simulink model "Pendulo"  (R2020b)
settings: Solver=FixedStepAuto  StartTime=0.0  StopTime=180  FixedStep=0.05  RelTol=1e-3
values from neighbouring files (symbols this model uses):
  g = 9.81    [PIDMiplanta.m]    (also in PID_Pendulo.m)
  l = 1.5    [PIDMiplanta.m]    (also in PID_Pendulo.m = 6.096)
  M = 583.756    [PIDMiplanta.m]    (also in PID_Pendulo.m)
  m = 116.7512    [PIDMiplanta.m]    (also in PID_Pendulo.m)
libraries: pid_lib x2, dspsrcs4 x1, commchan3 x1
settings Model: Creator=Matias  LastModifiedBy=Matias

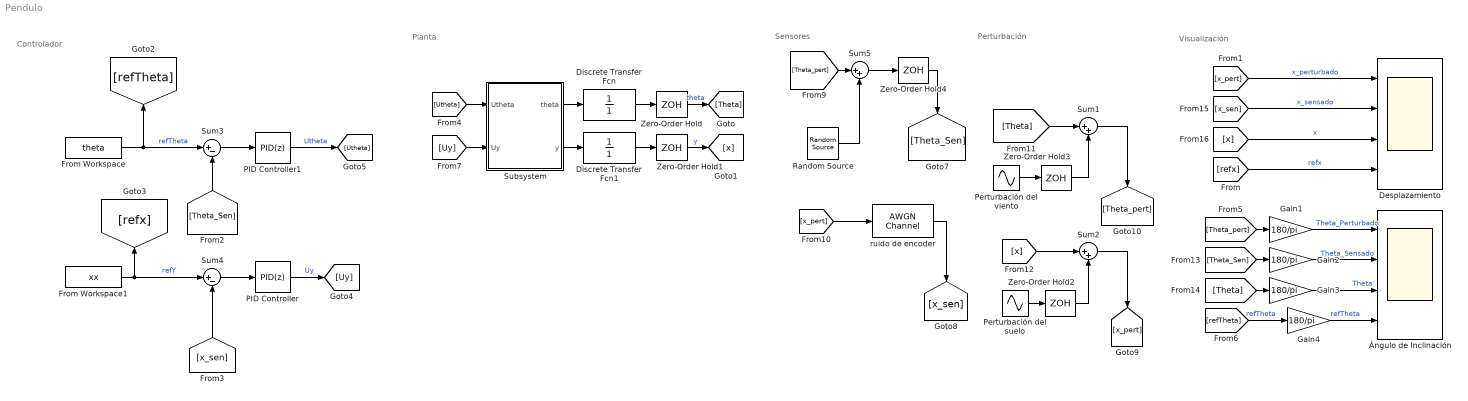
== system Pendulo ==
  note: Controlador
  note: Planta
  note: Perturbación
  note: Sensores
  note: Visualización
  Desplazamiento : Scope  NumInputPorts=4
  Discrete Transfer Fcn : DiscreteTransferFcn  Denominator=[1]
  Discrete Transfer Fcn1 : DiscreteTransferFcn  Denominator=[1]
  From Workspace : FromWorkspace  VariableName=theta
  From Workspace1 : FromWorkspace  VariableName=xx
  Gain{1..4} (4 alike) : Gain  Gain=180/pi
  PID Controller : pid_lib/PID Controller  Controller=PID  Form=Parallel  TimeDomain=Discrete-time  UseExternalTs=off  SampleTime=-1  IntegratorMethod=Forward Euler  FilterMethod=Forward Euler  ControllerParametersSource=internal  P=367.793686927  I=26.4785457931426  D=1277.18679492305  UseFilter=off  N=995.361556715437  TunerSelectOption=Transfer Function Based (PID Tuner App)  InitialConditionSource=internal  InitialConditionForIntegrator=0  InitialConditionForFilter=0  DifferentiatorICPrevScaledInput=0  ExternalReset=none  TrackingMode=off  Kt=1  LimitOutput=off  SatLimitsSource=internal  UpperSaturationLimit=inf  LowerSaturationLimit=-inf  LinearizeAsGain=on  AntiWindupMode=none  Kb=1  POutMin=[]  POutMax=[]  IOutMin=[]  IOutMax=[]  DOutMin=[]  DOutMax=[]  NOutMin=[]  NOutMax=[]  SumOutMin=[]  SumOutMax=[]  SaturationOutMin=[]  SaturationOutMax=[]  PParamMin=[]  PParamMax=[]  IParamMin=[]  IParamMax=[]  DParamMin=[]  DParamMax=[]  NParamMin=[]  NParamMax=[]  KbParamMin=[]  KbParamMax=[]  KtParamMin=[]  KtParamMax=[]  KbOutMin=[]  KbOutMax=[]  KtOutMin=[]  KtOutMax=[]  IntegratorOutMin=[]  IntegratorOutMax=[]  FilterOutMin=[]  FilterOutMax=[]  SumI1OutMin=[]  SumI1OutMax=[]  SumI2OutMin=[]  SumI2OutMax=[]  SumI3OutMin=[]  SumI3OutMax=[]  SumI4OutMin=[]  SumI4OutMax=[]  SumDOutMin=[]  SumDOutMax=[]  DifferentiatorOutMin=[]  DifferentiatorOutMax=[]  FilterDiffOutCoefMin=[]  FilterDiffOutCoefMax=[]  ReciprocalOutMin=[]  ReciprocalOutMax=[]  SumDenOutMin=[]  SumDenOutMax=[]  SumNumOutMin=[]  SumNumOutMax=[]  DivideOutMin=[]  DivideOutMax=[]  UdiffTsProdOutMin=[]  UdiffTsProdOutMax=[]  NTsProdOutMin=[]  NTsProdOutMax=[]  UintegralTsProdOutMin=[]  UintegralTsProdOutMax=[]  UngainTsProdOutMin=[]  UngainTsProdOutMax=[]  IntegratorContinuousStateAttributes=''  IntegratorStateMustResolveToSignalObject=off  IntegratorRTWStateStorageClass=Auto  FilterContinuousStateAttributes=''  FilterStateMustResolveToSignalObject=off  FilterRTWStateStorageClass=Auto  ParallelPVariant=InternalParameters  IdealPVariant=Disabled  IVariant=InternalParameters  DVariant=InternalParameters  IntegratorVariant=Discrete  SatVariant=Disabled  AWVariant=Passthrough  PCopyVariant=Disabled  TRVariant=Disabled  FdbkBlocksVariant=Forward  IdealPFdbkVariant=Disabled  SatFdbkVariant=Disabled  DerivativeFilterVariant=Differentiator  NVariant=Passthrough  NCopyVariant=Disabled_SignalSpec  FilterICVariant=InternalICsDifferentiator  IntegratorICVariant=InternalICs  ExternalResetVariant=Disabled  TRSumVariant=Passthrough  SumFdbkVariant=Disabled  SumVariant=Sum_PID  TsampFilterVariant=InternalTs  TsampNgainVariant=Passthrough  TsampIntegralVariant=Passthrough  ExternalSaturationOutDataTypeStr=Inherit: Same as second input
  PID Controller1 : pid_lib/PID Controller  Controller=PID  Form=Parallel  TimeDomain=Discrete-time  UseExternalTs=off  SampleTime=-1  IntegratorMethod=Forward Euler  FilterMethod=Forward Euler  ControllerParametersSource=internal  P=-2253.02199465803  I=-1255.49487156541  D=-1010.77834393764  UseFilter=off  N=38.4410251434361  TunerSelectOption=Transfer Function Based (PID Tuner App)  InitialConditionSource=internal  InitialConditionForIntegrator=0  InitialConditionForFilter=0  DifferentiatorICPrevScaledInput=0  ExternalReset=none  TrackingMode=off  Kt=1  LimitOutput=off  SatLimitsSource=internal  UpperSaturationLimit=inf  LowerSaturationLimit=-inf  LinearizeAsGain=on  AntiWindupMode=none  Kb=1  POutMin=[]  POutMax=[]  IOutMin=[]  IOutMax=[]  DOutMin=[]  DOutMax=[]  NOutMin=[]  NOutMax=[]  SumOutMin=[]  SumOutMax=[]  SaturationOutMin=[]  SaturationOutMax=[]  PParamMin=[]  PParamMax=[]  IParamMin=[]  IParamMax=[]  DParamMin=[]  DParamMax=[]  NParamMin=[]  NParamMax=[]  KbParamMin=[]  KbParamMax=[]  KtParamMin=[]  KtParamMax=[]  KbOutMin=[]  KbOutMax=[]  KtOutMin=[]  KtOutMax=[]  IntegratorOutMin=[]  IntegratorOutMax=[]  FilterOutMin=[]  FilterOutMax=[]  SumI1OutMin=[]  SumI1OutMax=[]  SumI2OutMin=[]  SumI2OutMax=[]  SumI3OutMin=[]  SumI3OutMax=[]  SumI4OutMin=[]  SumI4OutMax=[]  SumDOutMin=[]  SumDOutMax=[]  DifferentiatorOutMin=[]  DifferentiatorOutMax=[]  FilterDiffOutCoefMin=[]  FilterDiffOutCoefMax=[]  ReciprocalOutMin=[]  ReciprocalOutMax=[]  SumDenOutMin=[]  SumDenOutMax=[]  SumNumOutMin=[]  SumNumOutMax=[]  DivideOutMin=[]  DivideOutMax=[]  UdiffTsProdOutMin=[]  UdiffTsProdOutMax=[]  NTsProdOutMin=[]  NTsProdOutMax=[]  UintegralTsProdOutMin=[]  UintegralTsProdOutMax=[]  UngainTsProdOutMin=[]  UngainTsProdOutMax=[]  IntegratorContinuousStateAttributes=''  IntegratorStateMustResolveToSignalObject=off  IntegratorRTWStateStorageClass=Auto  FilterContinuousStateAttributes=''  FilterStateMustResolveToSignalObject=off  FilterRTWStateStorageClass=Auto  ParallelPVariant=InternalParameters  IdealPVariant=Disabled  IVariant=InternalParameters  DVariant=InternalParameters  IntegratorVariant=Discrete  SatVariant=Disabled  AWVariant=Passthrough  PCopyVariant=Disabled  TRVariant=Disabled  FdbkBlocksVariant=Forward  IdealPFdbkVariant=Disabled  SatFdbkVariant=Disabled  DerivativeFilterVariant=Differentiator  NVariant=Passthrough  NCopyVariant=Disabled_SignalSpec  FilterICVariant=InternalICsDifferentiator  IntegratorICVariant=InternalICs  ExternalResetVariant=Disabled  TRSumVariant=Passthrough  SumFdbkVariant=Disabled  SumVariant=Sum_PID  TsampFilterVariant=InternalTs  TsampNgainVariant=Passthrough  TsampIntegralVariant=Passthrough  ExternalSaturationOutDataTypeStr=Inherit: Same as second input
  Perturbación del suelo : Sin  Amplitude=0.001  Frequency=0.05  SampleTime=0
  Perturbación del viento : Sin  Amplitude=0.01  Frequency=0.07  SampleTime=0
  Random Source : dspsrcs4/Random Source  SrcType=Gaussian  NormMethod=Ziggurat  CltLength=12  MinVal=0  MaxVal=1  MeanVal=0  VarVal=var_Theta  RepMode=Not repeatable  rawSeed=1  IsInherit=off  SampMode=Discrete  SampTime=0.1  SampFrame=1  DataType=Double  OutComplex=Real  OutputFrames=off
  Subsystem : Subsystem
  Sum1 : Sum  Inputs=|++
  Sum2 : Sum  Inputs=|++
  Sum3 : Sum  Inputs=|+-
  Sum4 : Sum  Inputs=|+-
  Sum5 : Sum  Inputs=|++
  Zero-Order Hold{,1..4} (5 alike) : ZeroOrderHold  SampleTime=-1
  ruido de encoder : commchan3/AWGN Channel  InputProcessing=Columns as channels (frame based)  seed=67  noiseMode="Signal to noise ratio  (SNR)"  EbNodB=10  EsNodB=10  SNRdB=SNR_x  bitsPerSym=1  Ps=1  Tsym=1  variance=1
  Ángulo de Inclinación : Scope  NumInputPorts=4
  wires:
  From Workspace1/1 -> [refx], Sum4/1  "refY"
  Sum3/1 -> PID Controller1/1
  From Workspace/1 -> Sum3/1, [refTheta]  "refTheta"
  Sum4/1 -> PID Controller/1
  Discrete Transfer Fcn/1 -> Zero-Order Hold/1
  Subsystem/1(theta) -> Discrete Transfer Fcn/1
  Zero-Order Hold/1 -> [Theta]  "theta"
  Discrete Transfer Fcn1/1 -> Zero-Order Hold1/1
  Subsystem/2(y) -> Discrete Transfer Fcn1/1
  Zero-Order Hold1/1 -> [x]  "y"
  PID Controller1/1 -> [Utheta]  "Utheta"
  PID Controller/1 -> [Uy]  "Uy"
  [x_pert] -> Desplazamiento/1  "x_perturbado"
  Zero-Order Hold2/1 -> Sum2/2
  Zero-Order Hold4/1 -> [Theta_Sen]
  Perturbación del suelo/1 -> Zero-Order Hold2/1
  Perturbación del viento/1 -> Zero-Order Hold3/1
  [Theta_pert] -> Sum5/1
  Sum5/1 -> Zero-Order Hold4/1
  Random Source/1 -> Sum5/2
  [x_sen] -> Desplazamiento/2  "x_sensado"
  [x_pert] -> ruido de encoder/1
  [Theta] -> Gain3/1
  [x] -> Desplazamiento/3  "x"
  Gain2/1 -> Ángulo de Inclinación/2  "Theta_Sensado"
  [Theta] -> Sum1/1
  Gain3/1 -> Ángulo de Inclinación/3  "Theta"
  [Theta_pert] -> Gain1/1
  Gain1/1 -> Ángulo de Inclinación/1  "Theta_Perturbado"
  [Theta_Sen] -> Gain2/1
  Zero-Order Hold3/1 -> Sum1/2
  [x] -> Sum2/1
  Sum2/1 -> [x_pert]
  ruido de encoder/1 -> [x_sen]
  [refx] -> Desplazamiento/4  "refx"
  Sum1/1 -> [Theta_pert]
  [Theta_Sen] -> Sum3/2
  [x_sen] -> Sum4/2
  [refTheta] -> Gain4/1  "refTheta"
  Gain4/1 -> Ángulo de Inclinación/4  "refTheta"
  [Utheta] -> Subsystem/1(Utheta)
  [Uy] -> Subsystem/2(Uy)

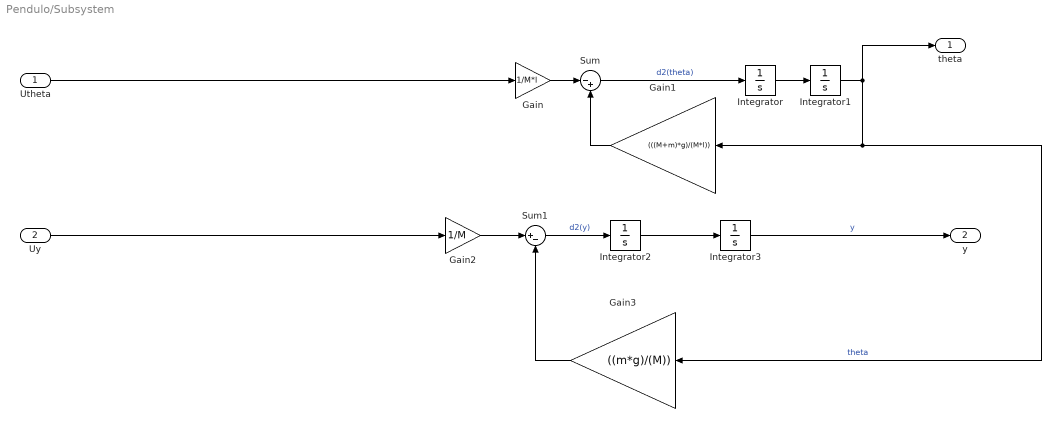
== system Pendulo/Subsystem ==
  Utheta : Inport
  Uy : Inport  Port=2
  Gain : Gain  Gain=1/M*l
  Gain1 : Gain  Gain=(((M+m)*g)/(M*l))
  Gain2 : Gain  Gain=1/M
  Gain3 : Gain  Gain=((m*g)/(M))
  Integrator{,1..3} (4 alike) : Integrator
  Sum : Sum  Inputs=|-+
  Sum1 : Sum  Inputs=|+-
  theta : Outport
  y : Outport  Port=2
  wires:
  Integrator2/1 -> Integrator3/1
  Gain/1 -> Sum/1
  Sum1/1 -> Integrator2/1  "d2(y)"
  Gain3/1 -> Sum1/2
  Gain1/1 -> Sum/2
  Gain2/1 -> Sum1/1
  Integrator/1 -> Integrator1/1
  Integrator1/1 -> Gain3/1, Gain1/1, theta/1  "theta"
  Sum/1 -> Integrator/1  "d2(theta)"
  Integrator3/1 -> y/1  "y"
  Utheta/1 -> Gain/1
  Uy/1 -> Gain2/1
